simulink model "STATCOM"  (R2024a)
settings: Solver=FixedStepDiscrete  StartTime=0.0  StopTime=0.4  FixedStep=Ts  RelTol=1e-3
InitFcn:
  | Ts=25e-6;
  | xInitial = STATCOMInit;
undefined symbols (not defined in the file or in its folder): DiscIntNeverNeededParam
libraries: spsThreeLevelBridgeLib x4, spsVoltageMeasurementLib x4, spsZigzagPhaseShiftingTransformerLib x4, spsThreePhaseVIMeasurementLib x3, spsDistributedParametersLineLib x3, spsSecondOrderFilterLib x3, spsSeriesRLCBranchLib x2, spsThreePhaseSourceLib x2, spsGroundLib x2, spsabctodq0Lib x2, spsThreePhaseSeriesRLCLoadLib x1, spsThreePhaseParallelRLCLoadLib x1
(part 1 of 3)
settings Model: FPTRunName=Active  Creator=The MathWorks, Inc.  LastModifiedBy=Monia
settings SolverCC: AlgebraicLoopSolver=TrustRegion
settings DataIOCC: LoadInitialState=on  SaveFinalState=on  SaveFormat=StructureWithTime  SaveOutput=off  SaveTime=off  ReturnWorkspaceOutputs=off  SignalLoggingName=sigsOut
settings OptimizationCC: BlockReduction=off  BooleanDataType=off  ExpressionDepthLimit=2147483647  InitFltsAndDblsToZero=on  EfficientMapNaN2IntZero=off  LifeSpan=inf
settings DebuggingCC: SaveWithParameterizedLinksMsg=none  UnderspecifiedInitializationDetection=Classic  MergeDetectMultiDrivingBlocksExec=none  CheckExecutionContextPreStartOutputMsg=on  SignalResolutionControl=TryResolveAllWithWarning  MultiTaskDSMMsg=warning  MultiTaskCondExecSysMsg=none  FcnCallInpInsideContextMsg=warning  UnconnectedInputMsg=warning  UnconnectedOutputMsg=warning  UnconnectedLineMsg=warning  StateNameClashWarn=warning  SubsystemReferenceDiagnosticForUnitTest=warning  SFUnexpectedBacktrackingDiag=warning  SFNoUnconditionalDefaultTransitionDiag=warning  SFExecutionAtInitializationDiag=none  ArithmeticOperatorsInVariantConditions=warning
settings HardwareCC: ProdBitPerPointer=32  ProdBitPerSizeT=32  ProdBitPerPtrDiffT=32  ProdLargestAtomicFloat=None  ProdIntDivRoundTo=Undefined  ProdEndianess=Unspecified  ProdWordSize=32  ProdHWDeviceType=32-bit Generic  TargetBitPerPointer=64  TargetBitPerSizeT=64  TargetBitPerPtrDiffT=64  TargetLongLongMode=on  TargetIntDivRoundTo=Zero  TargetEndianess=LittleEndian  TargetWordSize=64  TargetHWDeviceType=MATLAB Host  ProdEqTarget=off
settings ModelReferenceCC: EnableRefExpFcnMdlSchedulingChecks=on  PropagateSignalLabelsOutOfModel=off
settings SFSimCC: SimUseLocalCustomCode=off  CustomCodeUndefinedFunction=UseInterfaceOnly
settings RTWCC: RTWUseLocalCustomCode=off  GPUComputeCapability=3.5  DLArmComputeVersion=19.05
settings CodeAppCC: StateflowObjectComments=on
settings GRTTargetCC: TargetFcnLib=ansi_tfl_tmw.mat  TargetLangStandard=C89/C90 (ANSI)  CombineOutputUpdateFcns=off  MatFileLogging=off  GRTInterface=on
settings ConfigComp: CovMetricSettings=dw  CovSaveCumulativeToWorkspaceVar=on  CovSaveSingleToWorkspaceVar=on  CovExternalEMLEnable=off  CovSFcnEnable=off
settings SimscapeCC: SimscapeNormalizeSystem=off

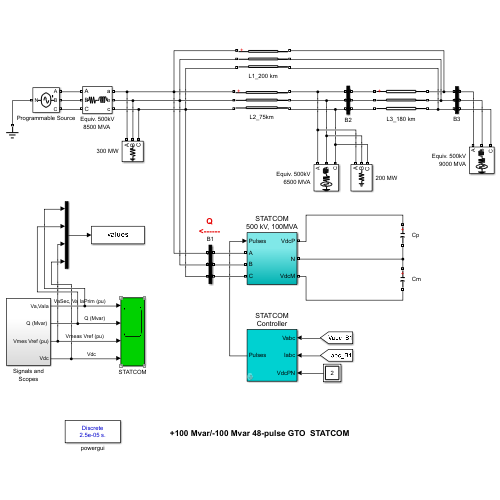
[thumbnail: Simulink's stored preview of the top-level diagram]
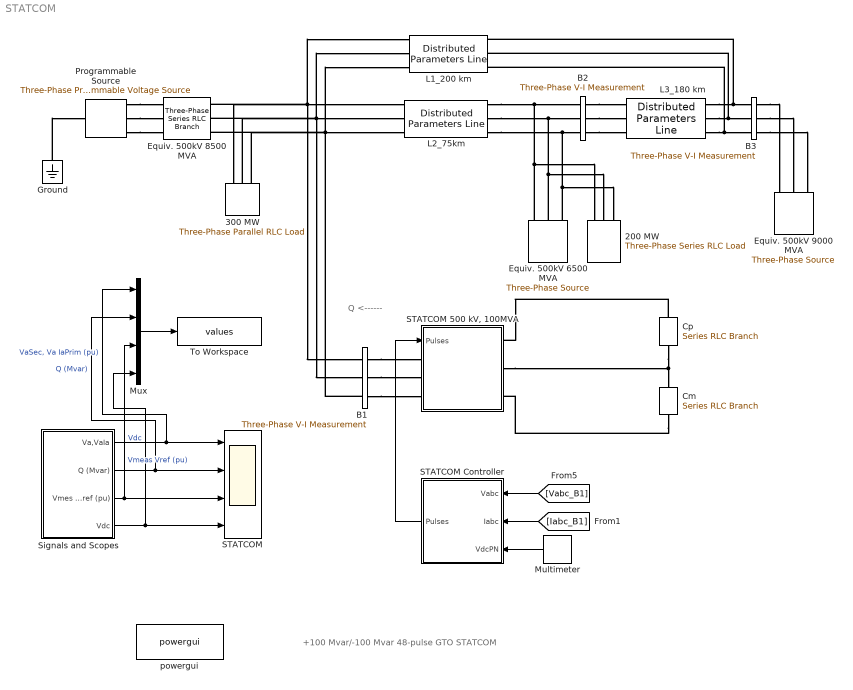
== system STATCOM ==
  note: Q
      | <------
  note: +100 Mvar/-100 Mvar 48-pulse GTO STATCOM
  200 MW : spsThreePhaseSeriesRLCLoadLib/Three-Phase Series RLC Load  LConnTagsString=A|B|C  Configuration=Y (grounded)  NominalVoltage=500e3  Vabc=[1e3 1e3 1e3]  Vabcp=[1e3 1e3 1e3]  NominalFrequency=60  UnbalancedPower=off  ActivePower=200e6  InductivePower=0  CapacitivePower=0  Pabc=[10e3 9e3 11e3]  QLabc=[100 90 110]  QCabc=[100 90 110]  Pabcp=[10e3 9e3 11e3]  QLabcp=[100 90 110]  QCabcp=[100 90 110]  Measurements=None  LoadType=constant Z
  300 MW : spsThreePhaseParallelRLCLoadLib/Three-Phase Parallel RLC Load  LConnTagsString=A|B|C  Configuration=Y (grounded)  NominalVoltage=500e3  Vabc=[1e3 1e3 1e3]  Vabcp=[1e3 1e3 1e3]  NominalFrequency=60  UnbalancedPower=off  ActivePower=300e6  InductivePower=0  CapacitivePower=0  Pabc=[10e3 9e3 11e3]  QLabc=[100 90 110]  QCabc=[100 90 110]  Pabcp=[10e3 9e3 11e3]  QLabcp=[100 90 110]  QCabcp=[100 90 110]  Measurements=None  LoadType=constant Z
  B1 : spsThreePhaseVIMeasurementLib/Three-Phase V-I Measurement  VoltageMeasurement=phase-to-ground  SetLabelV=on  LabelV=Vabc_B1  Vpu=on  VpuLL=off  CurrentMeasurement=yes  SetLabelI=on  LabelI=Iabc_B1  Ipu=on  Pbase=100e6  Vbase=500e3  OutputType=Magnitude  PhasorSimulation=off  PSBequivalent=0
  B2 : spsThreePhaseVIMeasurementLib/Three-Phase V-I Measurement  VoltageMeasurement=phase-to-ground  SetLabelV=on  LabelV=Vabc_B2  Vpu=on  VpuLL=off  CurrentMeasurement=no  SetLabelI=on  LabelI=Iabc_B3  Ipu=on  Pbase=100e6  Vbase=500e3  OutputType=Magnitude  PhasorSimulation=off  PSBequivalent=0
  B3 : spsThreePhaseVIMeasurementLib/Three-Phase V-I Measurement  VoltageMeasurement=phase-to-ground  SetLabelV=on  LabelV=Vabc_B3  Vpu=on  VpuLL=off  CurrentMeasurement=no  SetLabelI=on  LabelI=Iabc_B4  Ipu=on  Pbase=100e6  Vbase=500e3  OutputType=Magnitude  PhasorSimulation=off  PSBequivalent=0
  Cm : spsSeriesRLCBranchLib/Series RLC Branch  LConnTagsString=__new0  RConnTagsString=__new0  BranchType=C  Resistance=1.0  Inductance=1.0  SetiL0=off  InitialCurrent=0  Capacitance=3000e-6  Setx0=off  InitialVoltage=0  Measurements=Branch voltage
  Cp : spsSeriesRLCBranchLib/Series RLC Branch  LConnTagsString=__new0  RConnTagsString=__new0  BranchType=C  Resistance=1.0  Inductance=1.0  SetiL0=off  InitialCurrent=0  Capacitance=3000e-6  Setx0=off  InitialVoltage=0  Measurements=Branch voltage
  Equiv. 500kV 6500 MVA : spsThreePhaseSourceLib/Three-Phase Source  InternalConnection=Yg  VoltagePhases=off  Voltage=500e3*1.00  PhaseAngle=9.2-20  Voltage_phases=[25e3 25e3 25e3]/sqrt(3)  PhaseAngles_phases=[0 -120 +120]  Frequency=60  NonIdealSource=on  SpecifyImpedance=on  Resistance=0.8929  Inductance=16.58e-3  ShortCircuitLevel=6500e6  BaseVoltage=500e3  XRratio=8  BusType=swing  Pref=0  Qref=0  Prefabc=[10e3, 10e3, 10e3]  Qrefabc=[0, 0, 0]  Qmin=-inf  Qmax=inf
  "Equiv. 500kV 8500 MVA " : spsThreePhaseSeriesRLCBranchLib/Three-Phase Series RLC Branch  LConnTagsString=A|B|C  RConnTagsString=A|B|C  BranchType=RL  Resistance=500e3^2/8500e6/10  Inductance=500e3^2/8500e6/(2*pi*60)  Capacitance=inf  Measurements=None
  Equiv. 500kV 9000 MVA : spsThreePhaseSourceLib/Three-Phase Source  InternalConnection=Yg  VoltagePhases=off  Voltage=500e3*0.98  PhaseAngle=9.2-40  Voltage_phases=[25e3 25e3 25e3]/sqrt(3)  PhaseAngles_phases=[0 -120 +120]  Frequency=60  NonIdealSource=on  SpecifyImpedance=on  Resistance=0.8929  Inductance=16.58e-3  ShortCircuitLevel=9000e6  BaseVoltage=500e3  XRratio=10  BusType=swing  Pref=0  Qref=0  Prefabc=[10e3, 10e3, 10e3]  Qrefabc=[0, 0, 0]  Qmin=-inf  Qmax=inf
  Ground : spsGroundLib/Ground  LConnTagsString=a
  L1_200 km : spsDistributedParametersLineLib/Distributed Parameters Line  Phases=3  Length=200  Frequency=60  Resistance=[0.01273*2 0.3864]  Inductance="[0.9337e-3  4.1264e-3]"  Capacitance=[12.74e-9 7.751e-9]  x1=[-0.00115 -8.14287400104293e-11 2402.61943520303 -499904.221272758;-0.001125 -8.04202249960053e-11 7113.929264626 -499859.375261574;-0.0011 -7.94045665921992e-11 11824.6071937182 -499770.128850442;-0.001075 -7.83818550156633e-11 16534.2347928284 -499636.489966745;-0.00105 -7.73521811095532e-11 21242.3937256017 -499458.47048106;-0.001025 -7.63156363354588e-11 25948.6657861386 -499236.086206108;-0.001 -7.52723127652804e-11 30652.6329361427 -498969.356895346;-0.000975 -7.42223030730502e-11 35353.8773420527 -498658.306241214;-0.00095 -7.31657005267002e-11 40051.9814121576 -498302.961873029;-0.000925 -7.2102598979778e-11 44746.5278336888 -497903.355354533;-0.0009 -7.10330928631099e-11 49437.0996098889 -497459.522181087;-0.000875 -6.99572771764133e-11 54123.2800970515 -496971.50177652;-0.00085 -6.88752474798578e-11 58804.6530415295 -496439.337489626;-0.000825 -6.77870998855776e-11 63480.80261671 -495863.076590314;-0.0008 -6.66929310491338e-11 68151.3134599497 -495242.770265409;-0.000775 -6.55928381609289e-11 72815.7707094702 -494578.473614106;-0.00075 -6.44869189375742e-11 77473.7600412081 -493870.245643075;-0.000725 -6.33752716132097e-11 82124.8677056182 -493118.149261217;-0.0007 -6.22579949307782e-11 86768.6805644244 -492322.251274084;-0.000675 -6.11351881332551e-11 91404.7861273176 -491482.622377936;-0.00065 -6.00069509548321e-11 96032.7725885953 -490599.337153466;-0.000625 -5.88733836120591e-11 100652.228863741 -489672.474059176;-0.0006 -5.77345867949419e-11 105262.744625937 -488702.115424405;-0.000575 -5.65906616579984e-11 109863.910342516 -487688.347442017;-0.00055 -5.54417098112736e-11 114455.317311334 -486631.260160746;-0.000525 -5.42878333113137e-11 119036.557697076 -485530.947477196;-0.0005 -5.31291346521015e-11 123607.224567483 -484387.507127504;-0.000475 -5.19657167559514e-11 128166.911929494 -483201.04067865;-0.00045 -5.07976829643682e-11 132715.214765313 -481971.653519447;-0.000425 -4.96251370288667e-11 137251.729068384 -480699.45485117;-0.0004 -4.84481831017568e-11 141776.051879277 -479384.557677861;-0.000375 -4.72669257268915e-11 146287.781321477 -478027.078796289;-0.00035 -4.6081469830381e-11 150786.516637091 -476627.138785577;-0.000325 -4.48919207112726e-11 155271.858222434 -475184.861996493;-0.0003 -4.36983840321969e-11 159743.407663532 -473700.3765404;-0.000275 -4.25009658099831e-11 164200.767771508 -472173.814277879;-0.00025 -4.12997724062412e-11 168643.542617867 -470605.310807017;-0.000225 -4.00949105179148e-11 173071.337569655 -468995.005451363;-0.0002 -3.88864871678033e-11 177483.759324526 -467343.041247548;-0.000175 -3.7674609695056e-11 181880.415945663 -465649.564932585;-0.00015 -3.64593857456373e-11 186260.916896606 -463914.726930833;-0.000125 -3.52409232627648e-11 190624.873075931 -462138.681340632;-0.0001 -3.40193304773215e-11 194971.896851817 -460321.585920623;-7.5e-05 -3.2794715898242e-11 199301.602096478 -458463.602075727;-5e-05 -3.15671883028742e-11 203613.604220458 -456564.894842812;-2.5e-05 -3.03368567273166e-11 207907.520206798 -454625.632876033]  x2=[-0.00115 -1.23122642615639e-10 -128315.763299933 -475488.834003035;-0.001125 -1.21916356591108e-10 -123828.754086442 -476677.04584363;-0.0011 -1.20699241250852e-10 -119330.745687023 -477822.916472818;-0.001075 -1.19471404706093e-10 -114822.137640789 -478926.344107745;-0.00105 -1.18232956020373e-10 -110303.330428377 -479987.230735588;-0.001025 -1.16984005199864e-10 -105774.725436371 -481005.482122263;-0.001 -1.157246631836e-10 -101236.724921652 -481981.007820794;-0.000975 -1.1445504183362e-10 -96689.731975664 -482913.721179347;-0.00095 -1.13175253925034e-10 -92134.1504886127 -483803.53934893;-0.000925 -1.11885413136003e-10 -87570.385113586 -484650.383290748;-0.0009 -1.10585634037646e-10 -82998.8412306128 -485454.177783224;-0.000875 -1.09276032083856e-10 -78419.9249106538 -486214.851428684;-0.00085 -1.07956723601051e-10 -73834.0428795324 -486932.336659698;-0.000825 -1.06627825777839e-10 -69241.6024818066 -487606.569745078;-0.0008 -1.05289456654609e-10 -64643.0116445865 -488237.490795543;-0.000775 -1.03941735113044e-10 -60038.6788412997 -488825.043769038;-0.00075 -1.02584780865566e-10 -55429.0130554086 -489369.176475709;-0.000725 -1.01218714444695e-10 -50814.4237440817 -489869.840582544;-0.0007 -9.98436571923508e-11 -46195.3208018238 -490326.991617662;-0.000675 -9.84597312490685e-11 -41572.1145240663 -490740.588974265;-0.00065 -9.70670595431527e-11 -36945.2155707226 -491110.595914243;-0.000625 -9.56657657797567e-11 -32315.034929711 -491436.979571442;-0.0006 -9.42559744298952e-11 -27681.9838804482 -491719.710954577;-0.000575 -9.28378107193872e-11 -23046.4739573171 -491958.764949813;-0.00055 -9.14114006177337e-11 -18408.9169131121 -492154.12032299;-0.000525 -8.99768708269273e-11 -13769.7246824646 -492305.759721516;-0.0005 -8.85343487701988e-11 -9129.30934525293 -492413.669675903;-0.000475 -8.70839625806981e-11 -4488.08308999865 -492477.840600963;-0.00045 -8.56258410901127e-11 153.541822746251 -492498.266796665;-0.000425 -8.41601138172245e-11 4795.15309701867 -492474.946448636;-0.0004 -8.26869109564048e-11 9436.33843806696 -492407.881628323;-0.000375 -8.12063633660499e-11 14076.6855889733 -492297.078292812;-0.00035 -7.97186025569576e-11 18715.7823672728 -492142.546284297;-0.000325 -7.82237606806451e-11 23353.216701566 -491944.299329203;-0.0003 -7.67219705176114e-11 27988.576668121 -491702.355036971;-0.000275 -7.52133654655421e-11 32621.4505274637 -491416.734898492;-0.00025 -7.3698079527461e-11 37251.42676095 -491087.464284198;-0.000225 -7.21762472998266e-11 41878.0941073199 -490714.57244181;-0.0002 -7.06480039605766e-11 46501.0415992278 -490298.092493737;-0.000175 -6.91134852571211e-11 51119.8585997472 -489838.061434136;-0.00015 -6.75728274942839e-11 55734.1348388456 -489334.520125625;-0.000125 -6.60261675221958e-11 60343.4604498273 -488787.513295655;-0.0001 -6.44736427241384e-11 64947.4260057398 -488197.089532536;-7.5e-05 -6.29153910043412e-11 69545.6225557421 -487563.30128112;-5e-05 -6.13515507757319e-11 74137.6416614291 -486886.204838145;-2.5e-05 -5.97822609476419e-11 78723.0754331125 -486165.860347231]  x3=[-0.00115 4.29548969455391e-14 -16.7268516472353 53.7094281662912;-0.001125 3.7996422543363e-14 -17.2323007003137 53.5493982464096;-0.0011 3.30345730792374e-14 -17.736219080805 53.3846117593478;-0.001075 2.80697892933218e-14 -18.238562027765 53.2150833423944;-0.00105 2.31025121864187e-14 -18.7392849201884 53.0408280540435;-0.001025 1.81331829808022e-14 -19.2383432809728 52.8618613726575;-0.001 1.31622430810255e-14 -19.735692780869 52.6781991950918;-0.000975 8.19013403471294e-15 -20.2312892424186 52.4898578352829;-0.00095 3.21729749333921e-15 -20.7250886438783 52.2968540227995;-0.000925 -1.75582482700061e-15 -21.2170471231302 52.099204901356;-0.0009 -6.72879118482691e-15 -21.7071209815775 51.8969280272905;-0.000875 -1.17011598525137e-14 -22.1952666880264 51.6900413680043;-0.00085 -1.66724891555251e-14 -22.6814408825529 51.4785633003668;-0.000825 -2.16423375116476e-14 -23.1656003803538 51.2625126090827;-0.0008 -2.66102634702142e-14 -23.6477021755831 51.0419084850237;-0.000775 -3.15758257513162e-14 -24.1277034451717 50.8167705235236;-0.00075 -3.65385832850003e-14 -24.6055615526316 50.5871187226379;-0.000725 -4.14980952504474e-14 -25.0812340518425 50.3529734813675;-0.0007 -4.64539211151281e-14 -25.5546786908228 50.1143555978466;-0.000675 -5.14056206739341e-14 -26.025853415482 49.8712862674952;-0.00065 -5.63527540882795e-14 -26.4947163733567 49.6237870811367;-0.000625 -6.12948819251694e-14 -26.9612259173281 49.37188002308;-0.0006 -6.62315651962336e-14 -27.4253406093209 49.1155874691664;-0.000575 -7.11623653967194e-14 -27.8870192239848 48.8549321847826;-0.00055 -7.60868445444428e-14 -28.3462207523556 48.5899373228381;-0.000525 -8.1004565218692e-14 -28.8029044054985 48.3206264217086;-0.0005 -8.5915090599082e-14 -29.2570296181309 48.0470234031456;-0.000475 -9.08179845043552e-14 -29.7085560522255 47.7691525701512;-0.00045 -9.57128114311261e-14 -30.1574436005936 47.4870386048195;-0.000425 -1.00599136592565e-13 -30.6036523904478 47.2007065661442;-0.0004 -1.05476525957017e-13 -31.0471427869433 46.9101818877924;-0.000375 -1.10344546286557e-13 -31.4878753966988 46.6154903758459;-0.00035 -1.15202765175473e-13 -31.9258110712954 46.3166582065088;-0.000325 -1.20050751088673e-13 -32.3609109107545 46.0137119237822;-0.0003 -1.24888073400015e-13 -32.7931362669924 45.7066784371067;-0.000275 -1.29714302430563e-13 -33.2224487472539 45.3955850189718;-0.00025 -1.34529009486747e-13 -33.6488102175221 45.0804593024936;-0.000225 -1.39331766898449e-13 -34.0721828059061 44.7613292789605;-0.0002 -1.44122148056984e-13 -34.4925289060044 44.4382232953463;-0.000175 -1.48899727453e-13 -34.909811180246 44.1111700517928;-0.00015 -1.53664080714271e-13 -35.3239925632065 43.78019859906;-0.000125 -1.58414784643391e-13 -35.7350362649008 43.4453383359462;-0.0001 -1.6315141725537e-13 -36.1429057740504 43.1066190066761;-7.5e-05 -1.6787355781511e-13 -36.5475648613272 42.764070698259;-5e-05 -1.72580786874783e-13 -36.9489775825714 42.4177238378163;-2.5e-05 -1.77272686311086e-13 -37.347108281984 42.0676091898788]  x4=[-0.00115 -6.38756472573475e-13 -908.548219025938 -3545.71373384202;-0.001125 -6.49913175869781e-13 -875.090797843979 -3554.11899690766;-0.0011 -6.61012150119943e-13 -841.555646037492 -3562.20856257372;-0.001075 -6.72052409448893e-13 -807.945742392565 -3569.98171227821;-0.00105 -6.83032973196961e-13 -774.264072335175 -3577.43775556502;-0.001025 -6.93952866006985e-13 -740.513627666008 -3584.57603014527;-0.001 -7.04811117910944e-13 -706.697406294707 -3591.39590195615;-0.000975 -7.15606764416123e-13 -672.818411973584 -3597.89676521721;-0.00095 -7.26338846590775e-13 -638.879654030806 -3604.07804248418;-0.000925 -7.37006411149309e-13 -604.884147103091 -3609.93918470027;-0.0009 -7.47608510536961e-13 -570.834910867929 -3615.47967124495;-0.000875 -7.58144203013958e-13 -536.734969775358 -3620.69900998017;-0.00085 -7.68612552739178e-13 -502.587352779317 -3625.59673729407;-0.000825 -7.79012629853269e-13 -468.395093068592 -3630.1724181422;-0.0008 -7.89343510561247e-13 -434.161227797393 -3634.42564608613;-0.000775 -7.99604277214553e-13 -399.888797815577 -3638.35604332956;-0.00075 -8.09794018392566e-13 -365.580847398542 -3641.96326075188;-0.000725 -8.19911828983554e-13 -331.240423976816 -3645.24697793919;-0.0007 -8.29956810265079e-13 -296.870577865366 -3648.20690321273;-0.000675 -8.39928069983823e-13 -262.474361992656 -3650.84277365483;-0.00065 -8.49824722434843e-13 -228.05483162946 -3653.15435513223;-0.000625 -8.59645888540244e-13 -193.615044117482 -3655.1414423169;-0.0006 -8.69390695927266e-13 -159.158058597785 -3656.80385870428;-0.000575 -8.79058279005772e-13 -124.686935739055 -3658.14145662891;-0.00055 -8.88647779045133e-13 -90.2047374657405 -3659.15411727763;-0.000525 -8.98158344250508e-13 -55.7145266860712 -3659.84175070006;-0.0005 -9.07589129838506e-13 -21.2193670199947 -3660.20429581661;-0.000475 -9.1693929811222e-13 13.2776774729527 -3660.24172042394;-0.00045 -9.2620801853564e-13 47.7735425658145 -3659.95402119778;-0.000425 -9.35394467807427e-13 82.265164136394 -3659.34122369324;-0.0004 -9.44497829934038e-13 116.749478439429 -3658.40338234253;-0.000375 -9.53517296302213e-13 151.223422378733 -3657.14058045014;-0.00035 -9.62452065750798e-13 185.683933779272 -3655.55293018544;-0.000325 -9.71301344641908e-13 220.127951659169 -3653.64057257271;-0.0003 -9.80064346931425e-13 254.552416501598 -3651.40367747861;-0.000275 -9.88740294238818e-13 288.954270526545 -3648.84244359709;-0.00025 -9.9732841591628e-13 323.330457962422 -3645.95709843176;-0.000225 -1.00582794911719e-12 357.677925317494 -3642.74789827565;-0.0002 -1.01423813886386e-12 391.993621651109 -3639.21512818849;-0.000175 -1.02255823811461e-12 426.274498844702 -3635.35910197133;-0.00015 -1.03078750783011e-12 460.517511872547 -3631.18016213873;-0.000125 -1.03892521703905e-12 494.719619072228 -3626.67867988827;-0.0001 -1.04697064290305e-12 528.877782414824 -3621.85505506765;-7.5e-05 -1.05492307078085e-12 562.988967774763 -3616.70971613911;-5e-05 -1.06278179429184e-12 597.050145199325 -3611.2431201414;-2.5e-05 -1.07054611537874e-12 631.058289177786 -3605.45575264919]  x5=0.00113108313399148  V1=ones(3,3)  V2=ones(3,3)  I1=ones(3,3)  I2=ones(3,3)  nHarmo=1  Measurements=None  Decoupling=off  VsMag0=0  VrMag0=0  VsAngle0=0  VrAngle0=0  IsMag0=0  IrMag0=0  IsAngle0=0  IrAngle0=0
      settings: AttributesFormatString=\n
  L2_75km : spsDistributedParametersLineLib/Distributed Parameters Line  Phases=3  Length=75  Frequency=60  Resistance=[0.01273*2 0.3864]  Inductance="[0.9337e-3  4.1264e-3]"  Capacitance=[12.74e-9 7.751e-9]  x1=[-0.000425 -5.42682632567156e-11 0 0;-0.0004 -5.28203231777902e-11 0 0;-0.000375 -5.13676912923478e-11 0 0;-0.00035 -4.99104966315517e-11 0 0;-0.000325 -4.84488686318572e-11 0 0;-0.0003 -4.69829371235146e-11 0 0;-0.000275 -4.55128323190367e-11 164200.767771508 -472173.814277879;-0.00025 -4.40386848016324e-11 168643.542617867 -470605.310807017;-0.000225 -4.2560625513608e-11 173071.337569655 -468995.005451363;-0.0002 -4.10787857447356e-11 177483.759324526 -467343.041247548;-0.000175 -3.95932971205917e-11 181880.415945663 -465649.564932585;-0.00015 -3.81042915908652e-11 186260.916896606 -463914.726930833;-0.000125 -3.66119014176367e-11 190624.873075931 -462138.681340632;-0.0001 -3.51162591636306e-11 194971.896851817 -460321.585920623;-7.5e-05 -3.36174976804398e-11 199301.602096478 -458463.602075727;-5e-05 -3.21157500967254e-11 203613.604220458 -456564.894842812;-2.5e-05 -3.06111498063908e-11 207907.520206798 -454625.632876033]  x2=[-0.000425 -3.10526321174711e-11 0 0;-0.0004 -3.09596227976229e-11 0 0;-0.000375 -3.08638634650662e-11 0 0;-0.00035 -3.07653626256986e-11 0 0;-0.000325 -3.06641290289341e-11 0 0;-0.0003 -3.05601716669262e-11 0 0;-0.000275 -3.04534997737688e-11 117553.680103649 -485391.345094186;-0.00025 -3.03441228246764e-11 122123.097130952 -484261.886529797;-0.000225 -3.02320505351419e-11 126681.66647864 -483089.413024596;-0.0002 -3.01172928600741e-11 131228.983228225 -481874.028724459;-0.000175 -2.99998599929133e-11 135764.643460741 -480615.841586846;-0.00015 -2.98797623647257e-11 140288.24429262 -479314.963371214;-0.000125 -2.97570106432771e-11 144799.38391148 -477971.509629089;-0.0001 -2.96316157320851e-11 149297.661611816 -476585.599693799;-7.5e-05 -2.95035887694508e-11 153782.677830594 -475157.356669878;-5e-05 -2.93729411274693e-11 158254.03418274 -473686.907422131;-2.5e-05 -2.92396844110196e-11 162711.33349653 -472174.382564361]  x3=[-0.000425 1.24330745001038e-12 0 0;-0.0004 1.26230315164685e-12 0 0;-0.000375 1.28118672821863e-12 0 0;-0.00035 1.29995650237726e-12 0 0;-0.000325 1.31861080688287e-12 0 0;-0.0003 1.33714798475227e-12 0 0;-0.000275 1.35556638940615e-12 -105.220106231136 -45.9493438178069;-0.00025 1.37386438481529e-12 -104.782377150298 -46.9389645317315;-0.000225 1.39204034564596e-12 -104.33534069286 -47.9244158554206;-0.0002 1.4100926574042e-12 -103.879036567185 -48.9056102553896;-0.000175 1.42801971657932e-12 -103.413505304842 -49.8824605762786;-0.00015 1.44581993078626e-12 -102.938788257011 -50.8548800485938;-0.000125 1.46349171890707e-12 -102.454927590804 -51.822782296415;-0.0001 1.48103351123135e-12 -101.961966285524 -52.7860813450682;-7.5e-05 1.49844374959568e-12 -101.459948128844 -53.7446916287619;-5e-05 1.51572088752202e-12 -100.94891771292 -54.6985279981879;-2.5e-05 1.53286339035508e-12 -100.428920430428 -55.6475057280847]  x4=[-0.000425 -8.57991447070513e-13 0 0;-0.0004 -8.86924553394495e-13 0 0;-0.000375 -9.15778877951358e-13 0 0;-0.00035 -9.44551857733155e-13 0 0;-0.000325 -9.73240936957455e-13 0 0;-0.0003 -1.00184356729436e-12 0 0;-0.000275 -1.03035720809285e-12 968.495278147245 -3523.10319841842;-0.00025 -1.0587793266065e-12 1001.65623827972 -3513.81900939916;-0.000225 -1.08710739821838e-12 1034.72822551344 -3504.22270265824;-0.0002 -1.1153389066654e-12 1067.70830220326 -3494.31513059509;-0.000175 -1.14347134426172e-12 1100.59353886808 -3484.09717325757;-0.00015 -1.17150221212158e-12 1133.38101445104 -3473.56973826372;-0.000125 -1.19942902038121e-12 1166.06781657897 -3462.73376072119;-0.0001 -1.22724928842003e-12 1198.65104182112 -3451.59020314416;-7.5e-05 -1.25496054508098e-12 1231.12779594701 -3440.14005536784;-5e-05 -1.28256032889001e-12 1263.49519418355 -3428.38433446057;-2.5e-05 -1.31004618827473e-12 1295.7503614713 -3416.32408463345]  x5=0.000424156175246807  V1=ones(3,3)  V2=ones(3,3)  I1=ones(3,3)  I2=ones(3,3)  nHarmo=1  Measurements=None  Decoupling=off  VsMag0=0  VrMag0=0  VsAngle0=0  VrAngle0=0  IsMag0=0  IrMag0=0  IsAngle0=0  IrAngle0=0
      settings: AttributesFormatString=\n
  L3_180 km : spsDistributedParametersLineLib/Distributed Parameters Line  Phases=3  Length=180  Frequency=60  Resistance=[0.01273*2 0.3864]  Inductance="[0.9337e-3  4.1264e-3]"  Capacitance=[12.74e-9 7.751e-9]  x1=[-0.001025 -3.24420763710848e-11 -22533.8114980746 -498914.675007284;-0.001 -3.24169744920972e-11 -17830.7202854264 -499104.889790069;-0.000975 -3.23889931499971e-11 -13126.0452451034 -499250.771190669;-0.00095 -3.23581348302489e-11 -8420.20427354568 -499352.306251054;-0.000925 -3.23244022738672e-11 -3713.61537075788 -499409.485952292;-0.0009 -3.22877984771726e-11 993.303396819654 -499422.305215352;-0.000875 -3.22483266915259e-11 5700.13393344608 -499390.762901553;-0.00085 -3.22059904230394e-11 10406.4581512178 -499314.861812666;-0.000825 -3.21607934322653e-11 15111.8580072053 -499194.608690663;-0.0008 -3.21127397338615e-11 19815.9155405864 -499030.014217124;-0.000775 -3.20618335962356e-11 24518.2129097715 -498821.09301228;-0.00075 -3.20080795411649e-11 29218.3324295193 -498567.863633721;-0.000725 -3.19514823433954e-11 33915.8566080373 -498270.348574745;-0.0007 -3.18920470302174e-11 38610.3681840665 -497928.574262359;-0.000675 -3.18297788810193e-11 43301.4501639445 -497542.571054934;-0.00065 -3.17646834268179e-11 47988.6858586457 -497112.373239507;-0.000625 -3.1696766449768e-11 52671.6589207935 -496638.019028735;-0.0006 -3.16260339826482e-11 57349.9533816431 -496119.550557502;-0.000575 -3.15524923083251e-11 62023.1536880303 -495557.013879175;-0.00055 -3.14761479591954e-11 66690.8447392826 -494950.458961516;-0.000525 -3.13970077166059e-11 71352.6119240922 -494299.939682238;-0.0005 -3.13150786102502e-11 76008.0411573427 -493605.513824226;-0.000475 -3.12303679175455e-11 80656.7189168914 -492867.243070399;-0.00045 -3.11428831629852e-11 85298.2322803007 -492085.192998235;-0.000425 -3.10526321174711e-11 89932.1689615159 -491259.433073943;-0.0004 -3.09596227976229e-11 94558.1173474871 -490390.036646294;-0.000375 -3.08638634650662e-11 99175.666534731 -489477.080940105;-0.00035 -3.07653626256986e-11 103784.40636583 -488520.647049382;-0.000325 -3.06641290289341e-11 108383.927465863 -487520.819930112;-0.0003 -3.05601716669262e-11 112973.821278772 -486477.688392722;-0.000275 -3.04534997737688e-11 117553.680103649 -485391.345094186;-0.00025 -3.03441228246764e-11 122123.097130952 -484261.886529797;-0.000225 -3.02320505351419e-11 126681.66647864 -483089.413024596;-0.0002 -3.01172928600741e-11 131228.983228225 -481874.028724459;-0.000175 -2.99998599929133e-11 135764.643460741 -480615.841586846;-0.00015 -2.98797623647257e-11 140288.24429262 -479314.963371214;-0.000125 -2.97570106432771e-11 144799.38391148 -477971.509629089;-0.0001 -2.96316157320851e-11 149297.661611816 -476585.599693799;-7.5e-05 -2.95035887694508e-11 153782.677830594 -475157.356669878;-5e-05 -2.93729411274693e-11 158254.03418274 -473686.907422131;-2.5e-05 -2.92396844110196e-11 162711.33349653 -472174.382564361]  x2=[-0.001025 -1.16984005199864e-10 -105774.725436371 -481005.482122263;-0.001 -1.157246631836e-10 -101236.724921652 -481981.007820794;-0.000975 -1.1445504183362e-10 -96689.7319756641 -482913.721179347;-0.00095 -1.13175253925034e-10 -92134.1504886127 -483803.53934893;-0.000925 -1.11885413136003e-10 -87570.385113586 -484650.383290748;-0.0009 -1.10585634037646e-10 -82998.8412306128 -485454.177783224;-0.000875 -1.09276032083856e-10 -78419.9249106538 -486214.851428684;-0.00085 -1.07956723601051e-10 -73834.0428795324 -486932.336659698;-0.000825 -1.06627825777839e-10 -69241.6024818067 -487606.569745078;-0.0008 -1.05289456654609e-10 -64643.0116445865 -488237.490795543;-0.000775 -1.03941735113044e-10 -60038.6788412997 -488825.043769038;-0.00075 -1.02584780865566e-10 -55429.0130554086 -489369.176475709;-0.000725 -1.01218714444695e-10 -50814.4237440817 -489869.840582544;-0.0007 -9.98436571923508e-11 -46195.3208018238 -490326.991617662;-0.000675 -9.84597312490685e-11 -41572.1145240663 -490740.588974265;-0.00065 -9.70670595431527e-11 -36945.2155707226 -491110.595914243;-0.000625 -9.56657657797567e-11 -32315.034929711 -491436.979571442;-0.0006 -9.42559744298952e-11 -27681.9838804482 -491719.710954577;-0.000575 -9.28378107193872e-11 -23046.4739573171 -491958.764949813;-0.00055 -9.14114006177337e-11 -18408.9169131121 -492154.12032299;-0.000525 -8.99768708269273e-11 -13769.7246824646 -492305.759721516;-0.0005 -8.85343487701988e-11 -9129.30934525293 -492413.669675903;-0.000475 -8.70839625806981e-11 -4488.08308999865 -492477.840600963;-0.00045 -8.56258410901127e-11 153.541822746251 -492498.266796665;-0.000425 -8.41601138172245e-11 4795.15309701867 -492474.946448636;-0.0004 -8.26869109564048e-11 9436.33843806696 -492407.881628323;-0.000375 -8.12063633660499e-11 14076.6855889733 -492297.078292812;-0.00035 -7.97186025569576e-11 18715.7823672728 -492142.546284297;-0.000325 -7.82237606806451e-11 23353.216701566 -491944.299329203;-0.0003 -7.67219705176114e-11 27988.576668121 -491702.355036971;-0.000275 -7.52133654655421e-11 32621.4505274637 -491416.734898492;-0.00025 -7.3698079527461e-11 37251.42676095 -491087.464284198;-0.000225 -7.21762472998266e-11 41878.0941073199 -490714.57244181;-0.0002 -7.06480039605766e-11 46501.0415992278 -490298.092493737;-0.000175 -6.91134852571211e-11 51119.8585997472 -489838.061434136;-0.00015 -6.75728274942839e-11 55734.1348388456 -489334.520125625;-0.000125 -6.60261675221958e-11 60343.4604498273 -488787.513295655;-0.0001 -6.44736427241384e-11 64947.4260057398 -488197.089532536;-7.5e-05 -6.29153910043412e-11 69545.6225557421 -487563.30128112;-5e-05 -6.13515507757319e-11 74137.6416614291 -486886.204838145;-2.5e-05 -5.97822609476419e-11 78723.0754331125 -486165.860347231]  x3=[-0.001025 -4.58209043111222e-13 -109.121626749074 -481.83144086927;-0.001 -4.57739948981066e-13 -104.57569322624 -482.838473219329;-0.000975 -4.57230195741943e-13 -100.020470685667 -483.802617064376;-0.00095 -4.56679828673084e-13 -95.4563637485593 -484.723786763579;-0.000925 -4.56088896661273e-13 -90.883777825285 -485.601900493321;-0.0009 -4.55457452196509e-13 -86.3031190793651 -486.436880254462;-0.000875 -4.54785551367341e-13 -81.7147943913952 -487.228651879272;-0.00085 -4.54073253855884e-13 -77.1192113229044 -487.977145038018;-0.000825 -4.53320622932522e-13 -72.5167780801529 -488.682293245208;-0.0008 -4.52527725450286e-13 -67.9079034778729 -489.344033865502;-0.000775 -4.51694631838916e-13 -63.2929969029558 -489.962308119271;-0.00075 -4.50821416098601e-13 -58.6724682780873 -490.537061087823;-0.000725 -4.49908155793414e-13 -54.0467280253362 -491.068241718274;-0.0007 -4.48954932044415e-13 -49.4161870296983 -491.555802828089;-0.000675 -4.47961829522449e-13 -44.781256602599 -491.999701109273;-0.00065 -4.46928936440625e-13 -40.1423484453586 -492.399897132212;-0.000625 -4.45856344546479e-13 -35.4998746126222 -492.756355349182;-0.0006 -4.44744149113823e-13 -30.8542474757589 -493.069044097504;-0.000575 -4.43592448934288e-13 -26.2058796862324 -493.337935602354;-0.00055 -4.42401346308543e-13 -21.5551841389472 -493.563005979234;-0.000525 -4.4117094703721e-13 -16.9025739355724 -493.744235236093;-0.0005 -4.39901360411465e-13 -12.2484623478484 -493.881607275099;-0.000475 -4.38592699203336e-13 -7.59326278087678 -493.975109894074;-0.00045 -4.37245079655676e-13 -2.93738873639995 -494.024734787574;-0.000425 -4.35858621471846e-13 1.71874622392872 -494.03047754763;-0.0004 -4.34433447805079e-13 6.37472851527981 -493.992337664136;-0.000375 -4.3296968524754e-13 11.0301445663848 -493.910318524898;-0.00035 -4.31467463819083e-13 15.6845808562721 -493.784427415329;-0.000325 -4.29926916955701e-13 20.3376239509979 -493.614675517806;-0.0003 -4.28348181497675e-13 24.9888605403702 -493.401077910674;-0.000275 -4.26731397677416e-13 29.6378774746611 -493.143653566908;-0.00025 -4.25076709107011e-13 34.2842618013057 -492.842425352425;-0.000225 -4.23384262765468e-13 38.9276008015819 -492.497420024059;-0.0002 -4.21654208985655e-13 43.5674820272717 -492.108668227176;-0.000175 -4.19886701440953e-13 48.2034933372962 -491.67620449296;-0.00015 -4.18081897131602e-13 52.8352229343251 -491.200067235339;-0.000125 -4.16239956370757e-13 57.4622594013544 -490.680298747579;-0.0001 -4.14361042770245e-13 62.0841917382511 -490.116945198521;-7.5e-05 -4.12445323226038e-13 66.7006093982607 -489.510056628485;-5e-05 -4.10492967903421e-13 71.3111023244738 -488.859686944823;-2.5e-05 -4.08504150221883e-13 75.9152609862505 -488.16589391713]  x4=[-0.001025 2.38205280534021e-13 -780.765956967161 -3036.77016359515;-0.001 2.43519725295221e-13 -752.110820097334 -3043.99372869805;-0.000975 2.48812539226365e-13 -723.388876395687 -3050.94690867729;-0.00095 2.54083252189115e-13 -694.602677111331 -3057.62908591123;-0.000925 2.59331396008271e-13 -665.754779200931 -3064.03966685023;-0.0009 2.64556504513354e-13 -636.847745101581 -3070.17808206944;-0.000875 2.69758113580014e-13 -607.884142503195 -3076.04378631932;-0.00085 2.74935761171256e-13 -578.866544120424 -3081.63625857411;-0.000825 2.80088987378486e-13 -549.79752746414 -3086.95500207808;-0.0008 2.85217334462354e-13 -520.679674612482 -3091.99954438968;-0.000775 2.90320346893419e-13 -491.515571981502 -3096.7694374235;-0.00075 2.95397571392612e-13 -462.307810095427 -3101.26425749005;-0.000725 3.00448556971496e-13 -433.058983356549 -3105.48360533343;-0.0007 3.05472854972326e-13 -403.771689814779 -3109.42710616677;-0.000675 3.10470019107902e-13 -374.448530936871 -3113.09440970552;-0.00065 3.15439605501213e-13 -345.092111375346 -3116.48519019858;-0.000625 3.20381172724859e-13 -315.705038737132 -3119.59914645721;-0.0006 3.25294281840268e-13 -286.289923351938 -3122.43600188182;-0.000575 3.30178496436679e-13 -256.849378040396 -3124.9955044865;-0.00055 3.35033382669912e-13 -227.386017881967 -3127.27742692143;-0.000525 3.398585093009e-13 -197.902459982661 -3129.28156649308;-0.0005 3.44653447733995e-13 -168.401323242568 -3131.00774518217;-0.000475 3.49417772055042e-13 -138.88522812323 -3132.45580965953;-0.00045 3.54151059069206e-13 -109.356796414883 -3133.6256312997;-0.000425 3.58852888338566e-13 -79.8186510035658 -3134.51710619236;-0.0004 3.63522842219462e-13 -50.2734156381472 -3135.13015515156;-0.000375 3.68160505899585e-13 -20.7237146972657 -3135.46472372274;-0.00035 3.72765467434834e-13 8.82782704378189 -3135.52078218758;-0.000325 3.77337317785897e-13 38.378584646188 -3135.29832556666;-0.0003 3.81875650854593e-13 67.9259332407971 -3134.79737361985;-0.000275 3.86380063519936e-13 97.4672482612611 -3134.0179708446;-0.00025 3.90850155673949e-13 126.999905677169 -3132.96018647198;-0.000225 3.95285530257201e-13 156.521282227129 -3131.6241144605;-0.0002 3.99685793294074e-13 186.028755651779 -3130.00987348781;-0.000175 4.04050553927764e-13 215.519704926716 -3128.11760694013;-0.00015 4.08379424454992e-13 244.991510495304 -3125.94748289951;-0.000125 4.1267202036045e-13 274.441554501365 -3123.49969412892;-0.0001 4.16927960350949e-13 303.867221021706 -3120.7744580551;-7.5e-05 4.2114686638929e-13 333.265896298485 -3117.77201674929;-5e-05 4.25328363727844e-13 362.634968971378 -3114.49263690568;-2.5e-05 4.29472080941841e-13 391.971830309536 -3110.93660981775]  x5=0.00101797482059234  V1=ones(3,3)  V2=ones(3,3)  I1=ones(3,3)  I2=ones(3,3)  nHarmo=1  Measurements=None  Decoupling=off  VsMag0=0  VrMag0=0  VsAngle0=0  VrAngle0=0  IsMag0=0  IrMag0=0  IsAngle0=0  IrAngle0=0
      settings: AttributesFormatString=\n
  Multimeter : spsMultimeterLib/Multimeter  Tag=PoWeRsYsTeMmEaSuReMeNt  L=2  sel=[2 1]  yselected={}  Gain=[1 1]  OutputType=Magnitude  PlotAtSimulationStop=off  PhasorSimulation=off
      settings: AttributesFormatString=\n
  Mux : Mux
  Programmable Source : spsThreePhaseProgrammableVoltageSourceLib/Three-Phase Programmable Voltage Source  PositiveSequence="[500e3*1.0491 9.2  60]"  VariationEntity=Amplitude  VariationType=Table of time-amplitude pairs  VariationTypeAlt=Step  VariationStep=-0.3  VariationRate=0.5  VariationMagnitude=0.4  VariationFrequency=2  VariationTiming=[0.1 1.2]  VariationPhaseA=off  Amplitudes="[1  0.955  1.045  1 ]"  TimeValues=[0 0.1 0.2 0.3]  HarmonicGeneration=off  HarmonicA=[3 0.2 -25 0]  HarmonicB="[2 0.15  35 2]"  Timing="[0.1  0.6]"  BusType=swing  Pref=0  Qref=0  Qmin=-inf  Qmax=inf
  STATCOM : Scope  NumInputPorts=4
  "STATCOM 500 kV, 100MVA" : Subsystem
  STATCOM Controller : Subsystem  mask(STATCOM Controller){OpMode=Voltage regulation, Vref=1.0, Droop=0.03, Qref1=0, Iqref1=0, ParK_V=[12 3000], ParK_I=[5 40], Ts=Ts}
      mask prompts: OpMode "Operation Mode"; Vref "Reference voltage Vref (pu)"; Droop "Droop (pu/100 MVA):"; Qref1 "Reactive power setpoint Qref (pu)"; Iqref1 "Reactive current setpoint  Iqref (pu):"; ParK_V "Voltage regulator gains: [ Kp  Ki ]"; ParK_I "Iq regulator gains: [ Kp  Ki ]"; Ts "Sample time:"
      mask help:
      | This block implements a controller for a STATCOM using a 48-pulse inverter consisting of  four 3-level bridges and four phase-shifting transformers. The 'Pulses' output is a vectorized signal of the 48 pulses sent to the four 3-level inverters.
      | In Voltage control mode the primary voltage (Vabc) is controlled at Vref within the droop setting. In Var control mode, either the reactive power output or the reactive current is kept constant at Qref (Qref>0 for capacitive mode) or Iqref (Iqref>0 for capacitive mode) .
      mask init:
      | Kp_I=ParK_I(1);
      | Ki_I=ParK_I(2);
      | Kp_V=ParK_V(1);
      | Ki_V=ParK_V(2);
      mask TypeOptions OpMode: Voltage regulation | Var control (Fixed Qref) | Var control (Fixed Iqref)
  Signals and Scopes : Subsystem
  To Workspace : ToWorkspace  VariableName=values  SaveFormat=Timeseries  SampleTime=-1
  powergui : spspowerguiLib/powergui  Priority=2  SimulationMode=Discrete  SampleTime=Ts  frequency=60  Iterations=50  frequencyindice=60  Pbase=100e6  ErrMax=1e-4  UnitsV=kV  UnitsW=MW  buscounter=0  FunctionMessages=off  echomessages=off  EnableUseOfTLC=off  CurrentSourceSwitches=off  DisableSnubberDevices=off  DisableRonSwitches=off  DisableVfSwitches=off  DisplayEquations=off  AutomaticDiscreteSolvers=off  SolverType=Tustin/Backward Euler (TBE)  Interpol=off  ExternalGateDelay=off  methode=off  Ts=0  x0status=blocks  SPID=off  SwTol=0  HookPort=off  NonlinearTolerance=1e-4  nMaxIteration=100  ContinueOnMaxIteration=off  RestoreLinks=warning  ResistiveCurrentMeasurement=off  Frange=[0:2:500]  Ylog=off  Xlog=off  ShowGrid=off  save=off  variable=ZData  structure=VIstatcom  ZoomFFT=on  StartTime=0.3  cycles=1  DisplayStyle=off  fundamental=60  FreqAxis=on  MaxFrequency=4000  frequencyindicesteady=1  RmsSteady=1  display=off
  wires:
  Signals and Scopes/1(Va,VaIa) -> Mux/1, STATCOM/1  "VaSec, Va IaPrim (pu)"
  Signals and Scopes/2("Q (Mvar) ") -> Mux/2, STATCOM/2  "Q (Mvar)"
  Signals and Scopes/3(Vmes Vref (pu)) -> Mux/3, STATCOM/3  "Vmeas Vref (pu)"
  Signals and Scopes/4(Vdc) -> Mux/4, STATCOM/4  "Vdc"
  STATCOM Controller/1(Pulses) -> "STATCOM 500 kV, 100MVA"/1(Pulses)
  [Vabc_B1] -> STATCOM Controller/1(Vabc)
  [Iabc_B1] -> STATCOM Controller/2(Iabc)
  Multimeter/1 -> STATCOM Controller/3(VdcPN)
  Mux/1 -> To Workspace/1
  connections:
  Programmable Source/RConn1 -- "Equiv. 500kV 8500 MVA "/LConn1
  Programmable Source/RConn2 -- "Equiv. 500kV 8500 MVA "/LConn2
  Programmable Source/RConn3 -- "Equiv. 500kV 8500 MVA "/LConn3
  Equiv. 500kV 6500 MVA/RConn1 -- 200 MW/LConn1 -- L2_75km/RConn1 -- B2/LConn1
  Equiv. 500kV 6500 MVA/RConn2 -- 200 MW/LConn2 -- L2_75km/RConn2 -- B2/LConn2
  Equiv. 500kV 6500 MVA/RConn3 -- 200 MW/LConn3 -- L2_75km/RConn3 -- B2/LConn3
  300 MW/LConn2 -- "Equiv. 500kV 8500 MVA "/RConn2 -- L2_75km/LConn2 -- B1/LConn2 -- L1_200 km/LConn2
  B1/LConn3 -- 300 MW/LConn3 -- "Equiv. 500kV 8500 MVA "/RConn3 -- L2_75km/LConn3 -- L1_200 km/LConn3
  B2/RConn1 -- L3_180 km/LConn1
  B2/RConn2 -- L3_180 km/LConn2
  B2/RConn3 -- L3_180 km/LConn3
  "Equiv. 500kV 8500 MVA "/RConn1 -- 300 MW/LConn1 -- L2_75km/LConn1 -- B1/LConn1 -- L1_200 km/LConn1
  L3_180 km/RConn1 -- B3/LConn1 -- L1_200 km/RConn1
  L3_180 km/RConn2 -- B3/LConn2 -- L1_200 km/RConn2
  L3_180 km/RConn3 -- B3/LConn3 -- L1_200 km/RConn3
  B3/RConn1 -- Equiv. 500kV 9000 MVA/RConn1
  B3/RConn2 -- Equiv. 500kV 9000 MVA/RConn2
  B3/RConn3 -- Equiv. 500kV 9000 MVA/RConn3
  B1/RConn1 -- "STATCOM 500 kV, 100MVA"/LConn1
  B1/RConn2 -- "STATCOM 500 kV, 100MVA"/LConn2
  B1/RConn3 -- "STATCOM 500 kV, 100MVA"/LConn3
  Cp/LConn1 -- "STATCOM 500 kV, 100MVA"/RConn1
  Cm/RConn1 -- "STATCOM 500 kV, 100MVA"/RConn3
  Cp/RConn1 -- Cm/LConn1 -- "STATCOM 500 kV, 100MVA"/RConn2
  Ground/LConn1 -- Programmable Source/LConn1

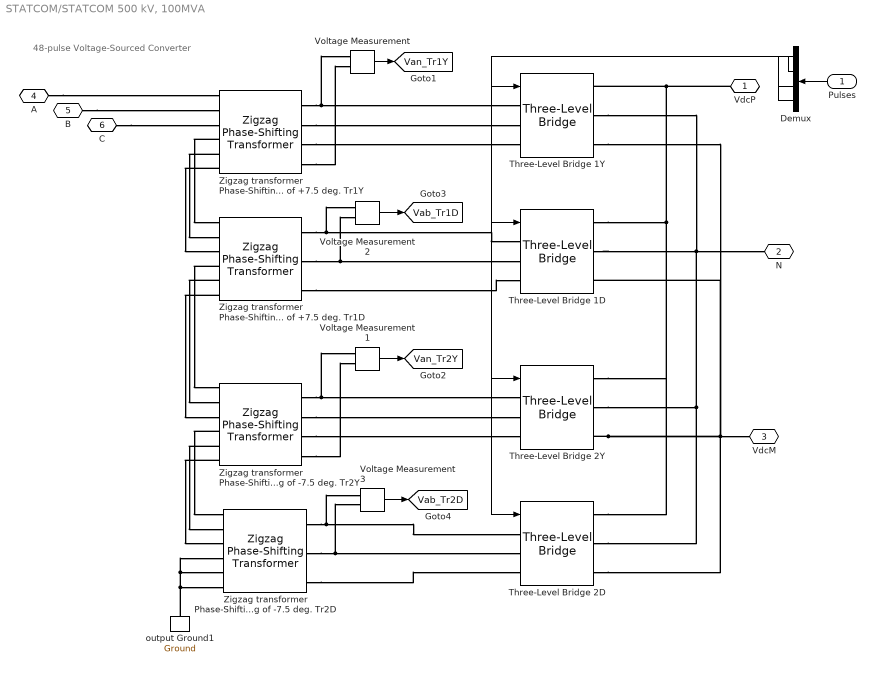
== system STATCOM/STATCOM 500 kV, 100MVA ==
  note: 48-pulse Voltage-Sourced Converter
  Pulses : Inport  PortDimensions=48
  Demux : Demux  Outputs=[12 12 12 12]
      settings: DisplayOption=none
  Three-Level Bridge 1D : spsThreeLevelBridgeLib/Three-Level Bridge  Arms=3  SnubberResistance=1e5  SbubberCapacitance=inf  Device=GTO / Diodes  Ron=1e-4  ForwardVoltages="[  0  0  ]"  Measurements=None
      settings: AttributesFormatString=\n
  Three-Level Bridge 1Y : spsThreeLevelBridgeLib/Three-Level Bridge  Arms=3  SnubberResistance=1e5  SbubberCapacitance=inf  Device=GTO / Diodes  Ron=1e-4  ForwardVoltages="[  0  0  ]"  Measurements=None
      settings: AttributesFormatString=\n
  Three-Level Bridge 2Y : spsThreeLevelBridgeLib/Three-Level Bridge  Arms=3  SnubberResistance=1e5  SbubberCapacitance=inf  Device=GTO / Diodes  Ron=1e-4  ForwardVoltages="[  0  0  ]"  Measurements=None
      settings: AttributesFormatString=\n
  Three-Level Bridge 2D : spsThreeLevelBridgeLib/Three-Level Bridge  Arms=3  SnubberResistance=1e5  SbubberCapacitance=inf  Device=GTO / Diodes  Ron=1e-4  ForwardVoltages="[  0  0  ]"  Measurements=None
      settings: AttributesFormatString=\n
  Voltage Measurement{,1..3} (4 alike) : spsVoltageMeasurementLib/Voltage Measurement  Tag=PoWeRsYsTeMmEaSuReMeNt  PhasorSimulation=off  OutputType=Magnitude  PSBequivalent=0
  Zigzag transformer Phase-Shifting of +7.5 deg. Tr1D : spsZigzagPhaseShiftingTransformerLib/Zigzag Phase-Shifting Transformer  SecondaryConnection=Delta D1(-30 deg.)  SetSaturation=off  SetInitialFlux=off  Measurements=None  UNITS=pu  NominalPower=[ 100e6/4 60]  PrimaryVoltage=500e3/4  SecondaryVoltage="[ 15e3  +7.5]"  Winding1=[ 0.05/30 0.05 ]  Winding2=[ 0.05/30 0.05 ]  Winding3=[ 0.05/30 0.05 ]  RmLm=[ 500 500 ]  Rm=500  Saturation=[ 0,0 ; 0.0024,1.2 ; 1.0,1.52 ]  InitialFluxes=[0,0,0]  BreakLoop=off  DiscreteSolver=Trapezoidal iterative  DataType=off
      settings: AttributesFormatString=\n
  Zigzag transformer Phase-Shifting of +7.5 deg. Tr1Y : spsZigzagPhaseShiftingTransformerLib/Zigzag Phase-Shifting Transformer  SecondaryConnection=Yn  SetSaturation=off  SetInitialFlux=off  Measurements=None  UNITS=pu  NominalPower=[ 100e6/4 60]  PrimaryVoltage=500e3/4  SecondaryVoltage="[ 15e3  +7.5]"  Winding1=[ 0.05/30 0.05 ]  Winding2=[ 0.05/30 0.05 ]  Winding3=[ 0.05/30 0.05 ]  RmLm=[ 500 500 ]  Rm=500  Saturation=[ 0,0 ; 0.0024,1.2 ; 1.0,1.52 ]  InitialFluxes=[0,0,0]  BreakLoop=off  DiscreteSolver=Trapezoidal iterative  DataType=off
      settings: AttributesFormatString=\n
  Zigzag transformer Phase-Shifting of -7.5 deg. Tr2D : spsZigzagPhaseShiftingTransformerLib/Zigzag Phase-Shifting Transformer  SecondaryConnection=Delta D1(-30 deg.)  SetSaturation=off  SetInitialFlux=off  Measurements=None  UNITS=pu  NominalPower=[ 100e6/4 60]  PrimaryVoltage=500e3/4  SecondaryVoltage="[ 15e3  -7.5]"  Winding1=[ 0.05/30 0.05 ]  Winding2=[ 0.05/30 0.05 ]  Winding3=[ 0.05/30 0.05 ]  RmLm=[ 500 500 ]  Rm=500  Saturation=[ 0,0 ; 0.0024,1.2 ; 1.0,1.52 ]  InitialFluxes=[0,0,0]  BreakLoop=off  DiscreteSolver=Trapezoidal iterative  DataType=off
      settings: AttributesFormatString=\n
  Zigzag transformer Phase-Shifting of -7.5 deg. Tr2Y : spsZigzagPhaseShiftingTransformerLib/Zigzag Phase-Shifting Transformer  SecondaryConnection=Yn  SetSaturation=off  SetInitialFlux=off  Measurements=None  UNITS=pu  NominalPower=[ 100e6/4 60]  PrimaryVoltage=500e3/4  SecondaryVoltage="[ 15e3  -7.5]"  Winding1=[ 0.05/30 0.05 ]  Winding2=[ 0.05/30 0.05 ]  Winding3=[ 0.05/30 0.05 ]  RmLm=[ 500 500 ]  Rm=500  Saturation=[ 0,0 ; 0.0024,1.2 ; 1.0,1.52 ]  InitialFluxes=[0,0,0]  BreakLoop=off  DiscreteSolver=Trapezoidal iterative  DataType=off
      settings: AttributesFormatString=\n
  output Ground1 : spsGroundLib/Ground  LConnTagsString=a  RConnTagsString=__newr0
  VdcP : PMIOPort  Side=Right
  N : PMIOPort  Port=2  Side=Right
  VdcM : PMIOPort  Port=3  Side=Right
  A : PMIOPort  Port=4  Side=Left
  B : PMIOPort  Port=5  Side=Left
  C : PMIOPort  Port=6  Side=Left
  tag scope: Vab_Tr1D=global, Vab_Tr2D=global, Van_Tr1Y=global, Van_Tr2Y=global
  wires:
  Pulses/1 -> Demux/1
  Voltage Measurement/1 -> [Van_Tr1Y]
  Voltage Measurement1/1 -> [Van_Tr2Y]
  Voltage Measurement2/1 -> [Vab_Tr1D]
  Voltage Measurement3/1 -> [Vab_Tr2D]
  Demux/1 -> Three-Level Bridge 1Y/1
  Demux/2 -> Three-Level Bridge 1D/1
  Demux/3 -> Three-Level Bridge 2Y/1
  Demux/4 -> Three-Level Bridge 2D/1
  connections:
  VdcP/RConn1 -- Three-Level Bridge 2Y/RConn1 -- Three-Level Bridge 2D/RConn1 -- Three-Level Bridge 1D/RConn1 -- Three-Level Bridge 1Y/RConn1
  Zigzag transformer Phase-Shifting of +7.5 deg. Tr1Y/RConn2 -- Three-Level Bridge 1Y/LConn2
  Zigzag transformer Phase-Shifting of +7.5 deg. Tr1Y/RConn3 -- Three-Level Bridge 1Y/LConn3
  Zigzag transformer Phase-Shifting of -7.5 deg. Tr2Y/RConn2 -- Three-Level Bridge 2Y/LConn2
  Zigzag transformer Phase-Shifting of -7.5 deg. Tr2Y/RConn3 -- Three-Level Bridge 2Y/LConn3
  Zigzag transformer Phase-Shifting of +7.5 deg. Tr1Y/RConn4 -- Voltage Measurement/LConn2
  Zigzag transformer Phase-Shifting of -7.5 deg. Tr2Y/RConn4 -- Voltage Measurement1/LConn2
  A/RConn1 -- Zigzag transformer Phase-Shifting of +7.5 deg. Tr1Y/LConn1
  B/RConn1 -- Zigzag transformer Phase-Shifting of +7.5 deg. Tr1Y/LConn2
  C/RConn1 -- Zigzag transformer Phase-Shifting of +7.5 deg. Tr1Y/LConn3
  Zigzag transformer Phase-Shifting of +7.5 deg. Tr1Y/LConn4 -- Zigzag transformer Phase-Shifting of +7.5 deg. Tr1D/LConn1
  Zigzag transformer Phase-Shifting of +7.5 deg. Tr1Y/LConn5 -- Zigzag transformer Phase-Shifting of +7.5 deg. Tr1D/LConn2
  Zigzag transformer Phase-Shifting of +7.5 deg. Tr1Y/LConn6 -- Zigzag transformer Phase-Shifting of +7.5 deg. Tr1D/LConn3
  Zigzag transformer Phase-Shifting of +7.5 deg. Tr1D/LConn4 -- Zigzag transformer Phase-Shifting of -7.5 deg. Tr2Y/LConn1
  Zigzag transformer Phase-Shifting of +7.5 deg. Tr1D/LConn5 -- Zigzag transformer Phase-Shifting of -7.5 deg. Tr2Y/LConn2
  Zigzag transformer Phase-Shifting of +7.5 deg. Tr1D/LConn6 -- Zigzag transformer Phase-Shifting of -7.5 deg. Tr2Y/LConn3
  Zigzag transformer Phase-Shifting of -7.5 deg. Tr2Y/LConn4 -- Zigzag transformer Phase-Shifting of -7.5 deg. Tr2D/LConn1
  Zigzag transformer Phase-Shifting of -7.5 deg. Tr2Y/LConn5 -- Zigzag transformer Phase-Shifting of -7.5 deg. Tr2D/LConn2
  Zigzag transformer Phase-Shifting of -7.5 deg. Tr2Y/LConn6 -- Zigzag transformer Phase-Shifting of -7.5 deg. Tr2D/LConn3
  output Ground1/LConn1 -- Zigzag transformer Phase-Shifting of -7.5 deg. Tr2D/LConn4 -- Zigzag transformer Phase-Shifting of -7.5 deg. Tr2D/LConn5 -- Zigzag transformer Phase-Shifting of -7.5 deg. Tr2D/LConn6
  Three-Level Bridge 2Y/RConn3 -- Three-Level Bridge 1Y/RConn3 -- Three-Level Bridge 1D/RConn3 -- Three-Level Bridge 2D/RConn3 -- VdcM/RConn1
  Zigzag transformer Phase-Shifting of +7.5 deg. Tr1D/RConn1 -- Three-Level Bridge 1D/LConn1 -- Voltage Measurement2/LConn1
  Zigzag transformer Phase-Shifting of +7.5 deg. Tr1D/RConn2 -- Three-Level Bridge 1D/LConn2 -- Voltage Measurement2/LConn2
  Zigzag transformer Phase-Shifting of +7.5 deg. Tr1D/RConn3 -- Three-Level Bridge 1D/LConn3
  Three-Level Bridge 2Y/RConn2 -- Three-Level Bridge 1D/RConn2 -- N/RConn1 -- Three-Level Bridge 1Y/RConn2 -- Three-Level Bridge 2D/RConn2
  Zigzag transformer Phase-Shifting of +7.5 deg. Tr1Y/RConn1 -- Three-Level Bridge 1Y/LConn1 -- Voltage Measurement/LConn1
  Zigzag transformer Phase-Shifting of -7.5 deg. Tr2Y/RConn1 -- Three-Level Bridge 2Y/LConn1 -- Voltage Measurement1/LConn1
  Zigzag transformer Phase-Shifting of -7.5 deg. Tr2D/RConn1 -- Three-Level Bridge 2D/LConn1 -- Voltage Measurement3/LConn1
  Zigzag transformer Phase-Shifting of -7.5 deg. Tr2D/RConn2 -- Three-Level Bridge 2D/LConn2 -- Voltage Measurement3/LConn2
  Zigzag transformer Phase-Shifting of -7.5 deg. Tr2D/RConn3 -- Three-Level Bridge 2D/LConn3
